simulink model "dongluchocnguoc"  (R2023b)
settings: Solver=FixedStepAuto  StartTime=0.0  StopTime=10  FixedStep=0.01  RelTol=1e-3
settings Model: Creator=DELL  LastModifiedBy=DELL

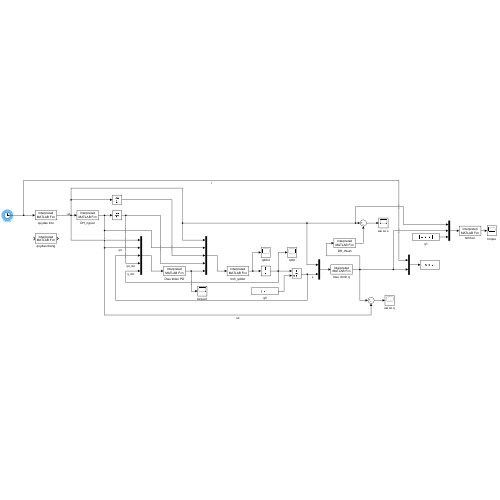
[thumbnail: Simulink's stored preview of the top-level diagram]
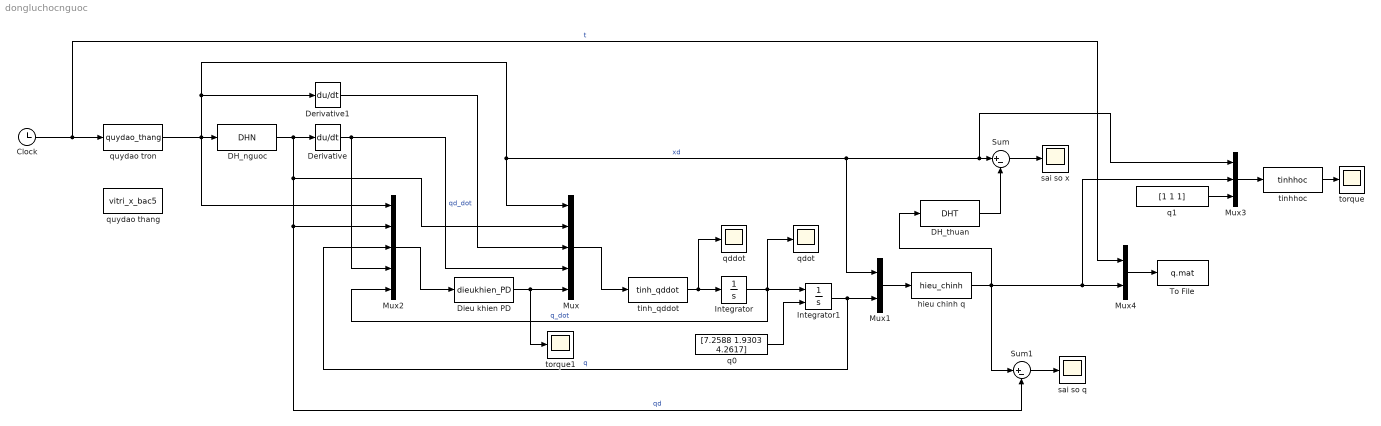
== system dongluchocnguoc ==
  Clock : Clock
      settings: Decimation=2
  DH_nguoc : MATLABFcn  MATLABFcn=DHN  OutputDimensions=3  OutputSignalType=real  Output1D=off
  DH_thuan : MATLABFcn  MATLABFcn=DHT  OutputDimensions=3  OutputSignalType=real  Output1D=off
  Derivative : Derivative
  Derivative1 : Derivative
  Dieu khien PD : MATLABFcn  MATLABFcn=dieukhien_PD  OutputDimensions=3  OutputSignalType=real  Output1D=off
  Integrator : Integrator
  Integrator1 : Integrator  InitialConditionSource=external
  Mux : Mux  Inputs=5
  Mux1 : Mux  Inputs=2
  Mux2 : Mux  Inputs=5
  Mux3 : Mux  Inputs=3
  Mux4 : Mux  Inputs=2
  Sum : Sum  Inputs=|+-
  Sum1 : Sum  Inputs=|+-
  To File : ToFile  Filename=q.mat  SaveFormat=Timeseries
  hieu chinh q : MATLABFcn  MATLABFcn=hieu_chinh  OutputDimensions=3  OutputSignalType=real  Output1D=off
  q0 : Constant  Value="[7.2588    1.9303    4.2617]"
  q1 : Constant  Value=[1 1 1]
  qddot : Scope
  qdot : Scope
  quydao thang : MATLABFcn  MATLABFcn=vitri_x_bac5  OutputDimensions=3
  quydao tron : MATLABFcn  MATLABFcn=quydao_thang  OutputDimensions=3
  sai so q : Scope
  sai so x : Scope
  tinh_qddot : MATLABFcn  MATLABFcn=tinh_qddot
  tinhhoc : MATLABFcn  MATLABFcn=tinhhoc  OutputDimensions=3  OutputSignalType=real  Output1D=off
  torque : Scope
  torque1 : Scope
  wires:
  Clock/1 -> Mux4/1, quydao tron/1  "t"
  quydao tron/1 -> Derivative1/1, Mux/1, Mux3/1, Sum/1, Mux1/1, Mux2/1, DH_nguoc/1  "xd"
  Mux/1 -> tinh_qddot/1
  Derivative/1 -> Mux/4, Mux2/4  "qd_dot"
  Dieu khien PD/1 -> torque1/1, Mux/5
  Integrator/1 -> Integrator1/1, qdot/1, Mux2/5  "q_dot"
  q0/1 -> Integrator1/2
  Integrator1/1 -> Mux1/2, Mux2/3  "q"
  Derivative1/1 -> Mux/3
  Mux2/1 -> Dieu khien PD/1
  DH_nguoc/1 -> Derivative/1, Mux2/2, Sum1/2, Mux/2  "qd"
  Sum/1 -> sai so x/1
  Sum1/1 -> sai so q/1
  DH_thuan/1 -> Sum/2
  Mux4/1 -> To File/1
  tinh_qddot/1 -> Integrator/1, qddot/1
  hieu chinh q/1 -> Mux3/2, Mux4/2, DH_thuan/1, Sum1/1
  Mux1/1 -> hieu chinh q/1
  Mux3/1 -> tinhhoc/1
  q1/1 -> Mux3/3
  tinhhoc/1 -> torque/1
